simulink model "FuzzyPidModel"  (R2015a)
settings: Solver=ode45  StartTime=0.0  StopTime=10.0  RelTol=1e-3
undefined symbols (not defined in the file or in its folder): Kdmax, Kdmin, Kpmax, Kpmin
libraries: fuzblock x1, simulink x1
settings Model: Creator=User  LastModifiedBy=User

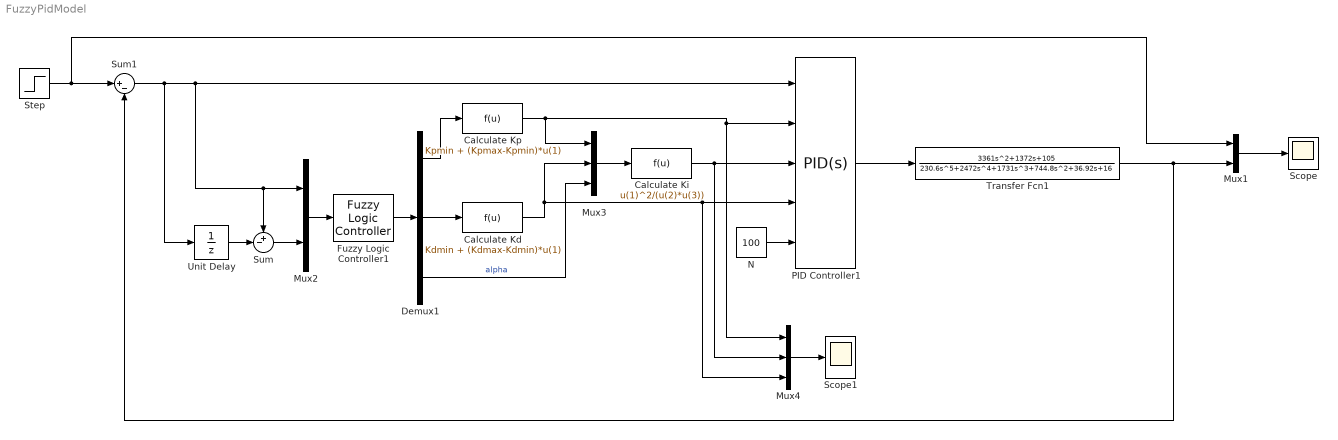
== system FuzzyPidModel ==
  Calculate Kd : Fcn  Expr=Kdmin + (Kdmax-Kdmin)*u(1)
  Calculate Ki : Fcn  Expr=u(1)^2/(u(2)*u(3))
  Calculate Kp : Fcn  Expr=Kpmin + (Kpmax-Kpmin)*u(1)
  Demux1 : Demux  Outputs=3
  Fuzzy Logic Controller1 : fuzblock/Fuzzy Logic  Controller  fis=fuzzy_pid
  Mux1 : Mux  Inputs=2
  Mux2 : Mux  Inputs=2
  Mux3 : Mux  Inputs=3
  Mux4 : Mux  Inputs=3
  N : Constant  Value=100
  PID Controller1 : simulink/Continuous/PID Controller  Controller=PID  TimeDomain=Continuous-time  SampleTime=-1  IntegratorMethod=Forward Euler  FilterMethod=Forward Euler  Form=Parallel  UseFilter=on  ControllerParametersSource=external  P=0.6*4.6737  I=1.2*4.6737/3.26  D=0.6*4.6737*3.26/8  N=100  InitialConditionSource=internal  InitialConditionForIntegrator=0  InitialConditionForFilter=0  ExternalReset=none  LimitOutput=off  UpperSaturationLimit=inf  LowerSaturationLimit=-inf  LinearizeAsGain=on  AntiWindupMode=none  Kb=1  TrackingMode=off  Kt=1  PParamMin=[]  PParamMax=[]  IParamMin=[]  IParamMax=[]  DParamMin=[]  DParamMax=[]  NParamMin=[]  NParamMax=[]  KbParamMin=[]  KbParamMax=[]  KtParamMin=[]  KtParamMax=[]  POutMin=[]  POutMax=[]  IOutMin=[]  IOutMax=[]  DOutMin=[]  DOutMax=[]  NOutMin=[]  NOutMax=[]  KbOutMin=[]  KbOutMax=[]  KtOutMin=[]  KtOutMax=[]  IntegratorOutMin=[]  IntegratorOutMax=[]  FilterOutMin=[]  FilterOutMax=[]  SumOutMin=[]  SumOutMax=[]  SumI1OutMin=[]  SumI1OutMax=[]  SumI2OutMin=[]  SumI2OutMax=[]  SumI3OutMin=[]  SumI3OutMax=[]  SumDOutMin=[]  SumDOutMax=[]  SaturationOutMin=[]  SaturationOutMax=[]  IntegratorContinuousStateAttributes=''  IntegratorStateMustResolveToSignalObject=off  IntegratorRTWStateStorageClass=Auto  FilterContinuousStateAttributes=''  FilterStateMustResolveToSignalObject=off  FilterRTWStateStorageClass=Auto  DifferentiatorICPrevScaledInput=0  DifferentiatorOutMin=[]  DifferentiatorOutMax=[]
  Scope : Scope
  Scope1 : Scope
  Step : Step  Time=0  SampleTime=0
  Sum : Sum  Inputs=+-|
  Sum1 : Sum  Inputs=|+-
  Transfer Fcn1 : TransferFcn  Numerator=[3361 1372 105]  Denominator=[230.6 2472 1731 744.8 36.92 16]
  Unit Delay : UnitDelay  SampleTime=-1
  wires:
  PID Controller1/1 -> Transfer Fcn1/1
  Sum1/1 -> Unit Delay/1, PID Controller1/1, Sum/1, Mux2/1
  N/1 -> PID Controller1/5
  Mux2/1 -> Fuzzy Logic Controller1/1
  Fuzzy Logic Controller1/1 -> Demux1/1
  Demux1/1 -> Calculate Kp/1
  Calculate Kp/1 -> Mux4/1, PID Controller1/2, Mux3/1
  Demux1/2 -> Calculate Kd/1
  Calculate Kd/1 -> Mux4/3, PID Controller1/4, Mux3/2
  Calculate Ki/1 -> Mux4/2, PID Controller1/3
  Mux3/1 -> Calculate Ki/1
  Sum/1 -> Mux2/2
  Unit Delay/1 -> Sum/2
  Mux4/1 -> Scope1/1
  Demux1/3 -> Mux3/3  "alpha"
  Transfer Fcn1/1 -> Sum1/2, Mux1/2
  Mux1/1 -> Scope/1
  Step/1 -> Mux1/1, Sum1/1
